simulink model "SMC_2WBR"  (R2017b)
settings: Solver=VariableStepAuto  StartTime=0.0  StopTime=10  RelTol=1e-3
settings Model: Creator=Iman  LastModifiedBy=Iman

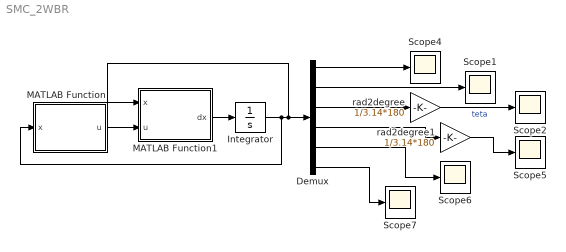
== system SMC_2WBR ==
  Demux : Demux  Outputs=6
  Integrator : Integrator  InitialCondition=[0;0;0;0;0;0]
  MATLAB Function : MATLAB Function  TreatAsAtomicUnit=on
  MATLAB Function1 : MATLAB Function  TreatAsAtomicUnit=on
  Scope{1..2,4..7} (6 alike) : Scope
  rad2degree : Gain  Gain=1/3.14*180
  rad2degree1 : Gain  Gain=1/3.14*180
  wires:
  MATLAB Function1/1(dx) -> Integrator/1
  Demux/1 -> Scope4/1
  rad2degree/1 -> Scope2/1  "teta"
  Demux/5 -> Scope6/1
  Demux/4 -> rad2degree1/1
  Demux/6 -> Scope7/1
  Demux/2 -> Scope1/1
  Integrator/1 -> MATLAB Function/1(x), Demux/1, MATLAB Function1/1(x)
  rad2degree1/1 -> Scope5/1
  Demux/3 -> rad2degree/1
  MATLAB Function/1(u) -> MATLAB Function1/2(u)

== matlab function SMC_2WBR/MATLAB Function1 ==
  data: x input; dx output; u input
function dx = fcn(x , u)
% 2wbr parameters---------------------------------------------------
d = 0.22;
l = 1.568e-2;
r = 2.75e-2;
Mb = 0.9;
Mw = 3.56e-2;
g = 9.81;
I1 = 4.564e-3;
I2 = 1.205e-3;
I3 = 3.879e-3;
J = 1.768e-5; 
K = 1.069e-5;
Ca = 0.25;
% dc motor parameters--------------------------------------------------
Km = 1.34;
Kb = 1;
R = 1.7;
L = 0.05;
J_m = 2.403e-5;  
J1 = 1.5842e-5;
N = 59;
% p.J_e = J1+N^2*J_m;
J_e = 2e-3;
B = 0.043;
% Equations
dx = x;
T = Km*x(6);
TR = T;
TL = T;

% assumed equations-------------------------------------------------
n1 = Mb+2*Mw+2*J/r^2;
n2 = Mb * l*cos(x(3));
n3 = -Mb*l*(x(6)^2+x(4)^2)*sin(x(3))+2/r*Ca*(x(2)/r-x(4))-(TR+TL)/r;
n4 = Mb*l*cos(x(3));
n5 = (I2+Mb*l^2);
n6 = (I3 - I1 - Mb*l^2)*x(6)^2*sin(x(3))*cos(x(3))-Mb*l*g*sin(x(3))-2*Ca*(x(2)/r-x(4))+(TL+TR);
n7 = (I3 + 2*K + Mw*d^2/2+J*d^2/r^2/2) -(I3 - I1 - Mb*l^2)*(sin(x(3)))^2;
n8 = (Mb*l*x(2)-2*(I3 - I1 - Mb*l^2)*x(4)*cos(x(3)))*x(6)*sin(x(3))+Ca*x(6)*d^2/r^2/2-(TR-TL)*d/2/r;

F1 = (n2*n6-n3*n5)/(n1*n5-n2*n4);
F2 = (n3*n4-n1*n6)/(n1*n5-n2*n4);
F3 = -n8/n7;

dx = [x(2); F1; x(4); F2;
    (T-B*x(5)+Ca*x(4))/J_e;
    (-Kb/L)*x(5)-R/L*x(6)+1/L*u];

== matlab function SMC_2WBR/MATLAB Function ==
  data: x input; u output
function u = fcn(x)
k=0.5;
s = x(4) + k*x(3);
u = -12*sign(s)-0.01;
end
